simulink model "simplifiedTV"  (R2020b)
settings: Solver=VariableStepAuto  StartTime=0.0  StopTime=10.0  RelTol=1e-3
undefined symbols (not defined in the file or in its folder): Car, Vec
libraries: simulink x4
settings Model: Creator=Isa  LastModifiedBy=Isa

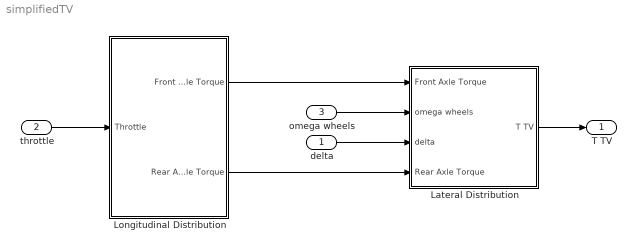
== system simplifiedTV ==
  delta : Inport
  "throttle " : Inport  Port=2
  omega wheels : Inport  Port=3
  Lateral Distribution : Subsystem
  Longitudinal Distribution : Subsystem
  T TV : Outport
  wires:
  Lateral Distribution/1(T TV) -> T TV/1
  Longitudinal Distribution/2(" Rear Axle Torque") -> Lateral Distribution/4(Rear Axle Torque)
  Longitudinal Distribution/1(Front Axle Torque) -> Lateral Distribution/1(Front Axle Torque)
  omega wheels/1 -> Lateral Distribution/2(omega wheels)
  delta/1 -> Lateral Distribution/3(delta)
  "throttle "/1 -> Longitudinal Distribution/1(Throttle)

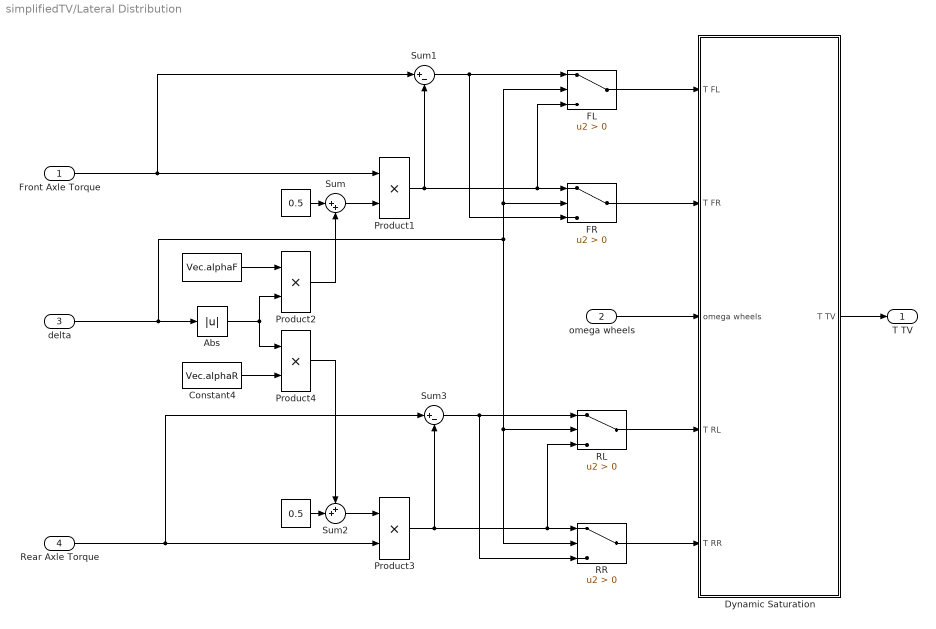
== system simplifiedTV/Lateral Distribution ==
  Front Axle Torque : Inport
  omega wheels : Inport  Port=2
  delta : Inport  Port=3
  Rear Axle Torque : Inport  Port=4
  " " : Constant  Value=Vec.alphaF
  "   " : Constant  Value=0.5
  " " : Constant  Value=0.5
  Abs : Abs
  Constant4 : Constant  Value=Vec.alphaR
  Dynamic Saturation : Subsystem
  FL : Switch  Criteria=u2 > Threshold
  FR : Switch  Criteria=u2 > Threshold
  Product{1..4} (4 alike) : Product
  RL : Switch  Criteria=u2 > Threshold
  RR : Switch  Criteria=u2 > Threshold
  Sum : Sum  Inputs=|++
  Sum1 : Sum  Inputs=|+-
  Sum2 : Sum  Inputs=++|
  Sum3 : Sum  Inputs=|+-
  T TV : Outport
  wires:
  Product3/1 -> Sum3/2, RL/3, RR/1
  Front Axle Torque/1 -> Product1/1, Sum1/1
  Sum3/1 -> RR/3, RL/1
  delta/1 -> Abs/1, RR/2, RL/2, FL/2, FR/2
  " "/1 -> Product2/1
  Sum1/1 -> FR/3, FL/1
  Product1/1 -> Sum1/2, FL/3, FR/1
  Product2/1 -> Sum/2
  "   "/1 -> Sum2/2
  Rear Axle Torque/1 -> Product3/2, Sum3/1
  Product4/1 -> Sum2/1
  " "/1 -> Sum/1
  Sum/1 -> Product1/2
  Abs/1 -> Product4/1, Product2/2
  Sum2/1 -> Product3/1
  Constant4/1 -> Product4/2
  FL/1 -> Dynamic Saturation/1(T FL)
  FR/1 -> Dynamic Saturation/2(T FR)
  omega wheels/1 -> Dynamic Saturation/3(omega wheels)
  RL/1 -> Dynamic Saturation/4(T RL)
  RR/1 -> Dynamic Saturation/5(T RR)
  Dynamic Saturation/1(T TV) -> T TV/1

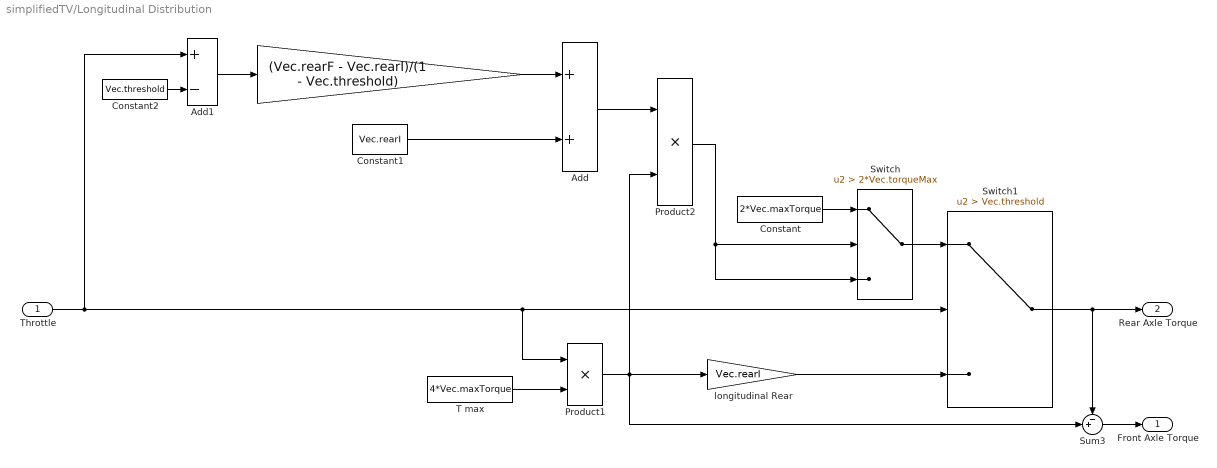
== system simplifiedTV/Longitudinal Distribution ==
  Throttle : Inport
  " " : Gain  Gain=(Vec.rearF - Vec.rearI)/(1 - Vec.threshold)
  Add : Sum
  Add1 : Sum  Inputs=+-
  Constant : Constant  Value=2*Vec.maxTorque
  Constant1 : Constant  Value=Vec.rearI
  Constant2 : Constant  Value=Vec.threshold
  Product1 : Product
  Product2 : Product
  Sum3 : Sum  Inputs=-+|
  Switch : Switch  Criteria=u2 > Threshold  Threshold=2*Vec.torqueMax
  Switch1 : Switch  Criteria=u2 > Threshold  Threshold=Vec.threshold
  "T max " : Constant  Value=4*Vec.maxTorque
  longitudinal Rear : Gain  Gain=Vec.rearI
  Front Axle Torque : Outport
  " Rear Axle Torque" : Outport  Port=2
  wires:
  "T max "/1 -> Product1/2
  Product2/1 -> Switch/2, Switch/3
  Add1/1 -> " "/1
  Constant1/1 -> Add/2
  longitudinal Rear/1 -> Switch1/3
  " "/1 -> Add/1
  Switch1/1 -> Sum3/1, " Rear Axle Torque"/1
  Throttle/1 -> Switch1/2, Product1/1, Add1/1
  Add/1 -> Product2/1
  Switch/1 -> Switch1/1
  Product1/1 -> Sum3/2, Product2/2, longitudinal Rear/1
  Constant2/1 -> Add1/2
  Constant/1 -> Switch/1
  Sum3/1 -> Front Axle Torque/1

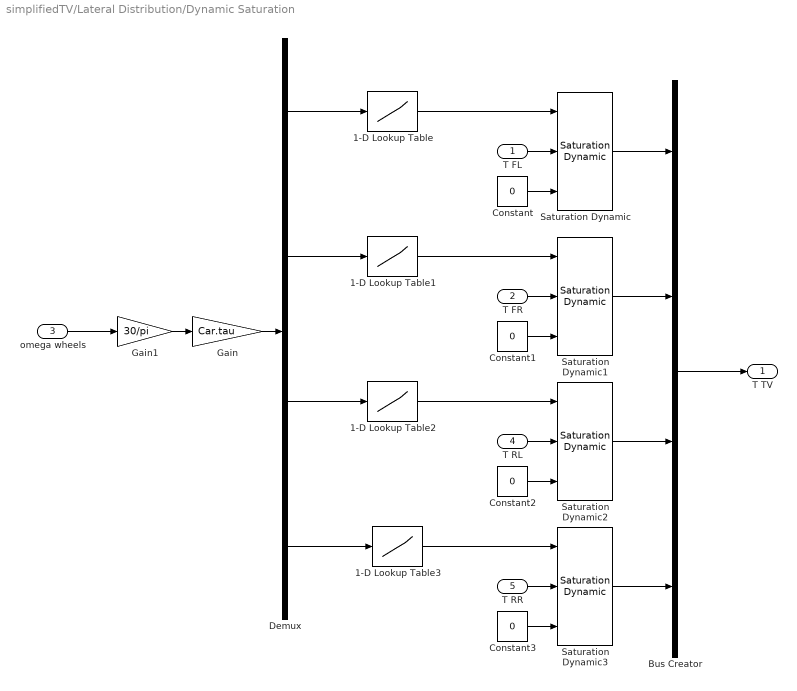
== system simplifiedTV/Lateral Distribution/Dynamic Saturation ==
  T FL : Inport
  T FR : Inport  Port=2
  omega wheels : Inport  Port=3
  T RL : Inport  Port=4
  T RR : Inport  Port=5
  1-D Lookup Table{,1..3} (4 alike) : Lookup_n-D  NumberOfTableDimensions=1  BreakpointsForDimension1=Car.rpm  Table=Car.torque  InternalRulePriority=Speed  RndMeth=Simplest  InputSameDT=on
  Bus Creator : BusCreator  Inputs=4
  Constant{,1..3} (4 alike) : Constant  Value=0
  Demux : Demux
  Gain : Gain  Gain=Car.tau
  Gain1 : Gain  Gain=30/pi
  Saturation Dynamic{,1..3} (4 alike) : simulink/Discontinuities/Saturation Dynamic  OutMin=[]  OutMax=[]  OutDataTypeStr=Inherit: Same as second input  OutDataType=fixdt(1, 16)  OutScaling=2^-10  DoSatur=off
  T TV : Outport
  wires:
  Demux/1 -> 1-D Lookup Table/1
  Saturation Dynamic/1 -> Bus Creator/1
  Constant3/1 -> Saturation Dynamic3/3
  1-D Lookup Table2/1 -> Saturation Dynamic2/1
  Gain/1 -> Demux/1
  Demux/3 -> 1-D Lookup Table2/1
  Saturation Dynamic3/1 -> Bus Creator/4
  Gain1/1 -> Gain/1
  Demux/4 -> 1-D Lookup Table3/1
  Saturation Dynamic1/1 -> Bus Creator/2
  1-D Lookup Table/1 -> Saturation Dynamic/1
  Constant2/1 -> Saturation Dynamic2/3
  1-D Lookup Table3/1 -> Saturation Dynamic3/1
  Constant1/1 -> Saturation Dynamic1/3
  1-D Lookup Table1/1 -> Saturation Dynamic1/1
  Saturation Dynamic2/1 -> Bus Creator/3
  Constant/1 -> Saturation Dynamic/3
  Demux/2 -> 1-D Lookup Table1/1
  omega wheels/1 -> Gain1/1
  T RL/1 -> Saturation Dynamic2/2
  Bus Creator/1 -> T TV/1
  T RR/1 -> Saturation Dynamic3/2
  T FL/1 -> Saturation Dynamic/2
  T FR/1 -> Saturation Dynamic1/2
